simulink model "PROJECTQ4"  (R2022a)
settings: Solver=VariableStepAuto  StartTime=0.0  StopTime=10.0  RelTol=1e-3
settings Model: Creator=1234567890  LastModifiedBy=1234567890

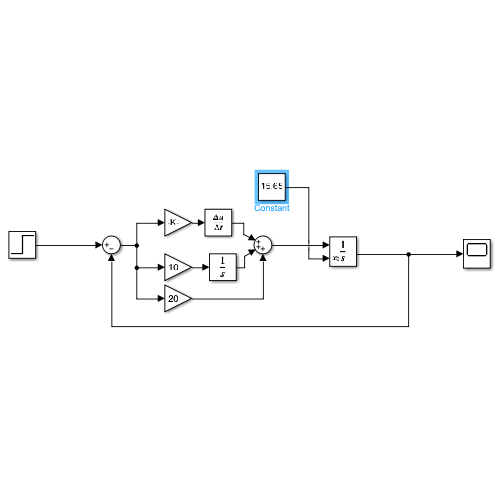
[thumbnail: Simulink's stored preview of the top-level diagram]
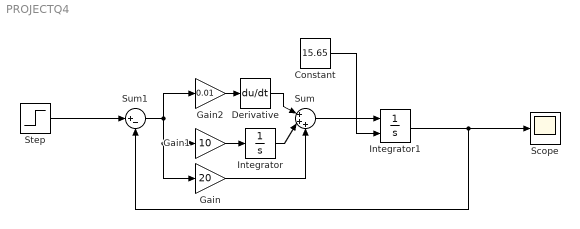
== system PROJECTQ4 ==
  Constant : Constant  Value=15.65
  Derivative : Derivative
  Gain : Gain  Gain=20
  Gain1 : Gain  Gain=10
  Gain2 : Gain  Gain=0.01
  Integrator : Integrator
  Integrator1 : Integrator  InitialConditionSource=external
  Scope : Scope
  Step : Step  Time=0  Before=15.65  After=15.65  SampleTime=0
  Sum : Sum  Inputs=|+++
  Sum1 : Sum  Inputs=|+-
  wires:
  Sum/1 -> Integrator1/1
  Gain/1 -> Sum/3
  Sum1/1 -> Gain2/1, Gain1/1, Gain/1
  Gain2/1 -> Derivative/1
  Gain1/1 -> Integrator/1
  Derivative/1 -> Sum/1
  Integrator/1 -> Sum/2
  Integrator1/1 -> Scope/1, Sum1/2
  Step/1 -> Sum1/1
  Constant/1 -> Integrator1/2
